simulink model "example_WeatherDatafile"  (R2016b)
settings: Solver=ode45  StartTime=0.0  StopTime=24*3600  RelTol=1e-3  EnableMultiTasking=on
libraries: carnot x2
settings Model: Creator=drhf  LastModifiedBy=drhf
settings DataIOCC: LimitDataPoints=on  SaveFormat=Array
settings OptimizationCC: ExpressionDepthLimit=2147483647  LifeSpan=inf
settings DebuggingCC: UnderspecifiedInitializationDetection=Classic  MergeDetectMultiDrivingBlocksExec=none  StateNameClashWarn=warning  SFUnexpectedBacktrackingDiag=warning  SFNoUnconditionalDefaultTransitionDiag=warning  SFExecutionAtInitializationDiag=none
settings HardwareCC: ProdBitPerPointer=32  ProdBitPerSizeT=32  ProdBitPerPtrDiffT=32  ProdLargestAtomicFloat=None  ProdIntDivRoundTo=Undefined  ProdEndianess=Unspecified  ProdWordSize=32  ProdHWDeviceType=32-bit Generic
settings ModelReferenceCC: PropagateSignalLabelsOutOfModel=off
settings GRTTargetCC: TargetLangStandard=C89/C90 (ANSI)  GeneratePreprocessorConditionals=Disable all  CombineOutputUpdateFcns=off  GRTInterface=on
settings ConfigComp: CovMetricSettings=dw  CovHtmlReporting=on  CovSaveCumulativeToWorkspaceVar=on  CovSaveSingleToWorkspaceVar=on  CovExternalEMLEnable=off

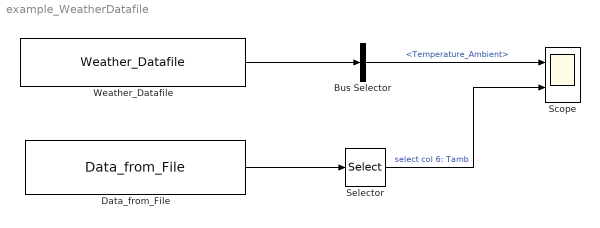
== system example_WeatherDatafile ==
  Bus Selector : BusSelector  OutputSignals=Temperature_Ambient
  Data_from_File : carnot/Load/General/Data_from_File  PathName='C:\repos\carnot_svn\trunk\public\data\'  FileName='DE_TRY2010_01_extremeWinter.mat'  UserParam=off  VariableName=DE_TRY2010_01_extremeWinter  SampleTime=3600
  Scope : Scope  NumInputPorts=2
  Selector : Selector  InputPortWidth=18  IndexOptions=Index vector (dialog)  Indices=[6]  OutputSizes=1
  Weather_Datafile : carnot/Weather/Weather_Datafile  PathName='C:\repos\carnot_svn\trunk\public\data\'  FileName='DE_TRY2010_01_extremeWinter.mat'  UserParam=off  VariableName=DE_TRY2010_01_extremeWinter  SampleTime=3600
  wires:
  Weather_Datafile/1 -> Bus Selector/1
  Bus Selector/1 -> Scope/1  "<Temperature_Ambient>"
  Data_from_File/1 -> Selector/1
  Selector/1 -> Scope/2  "select col 6: Tamb"
